simulink model "m04_linearization_model"  (R2021a)
settings: Solver=VariableStepAuto  StartTime=0.0  StopTime=10  RelTol=1e-3
undefined symbols (not defined in the file or in its folder): a, b, Cf, Cq, Cr, hs, Ix, Iz, Kq, M, ms
libraries: simulink x2
settings Model: Creator=jaime  LastModifiedBy=jaime

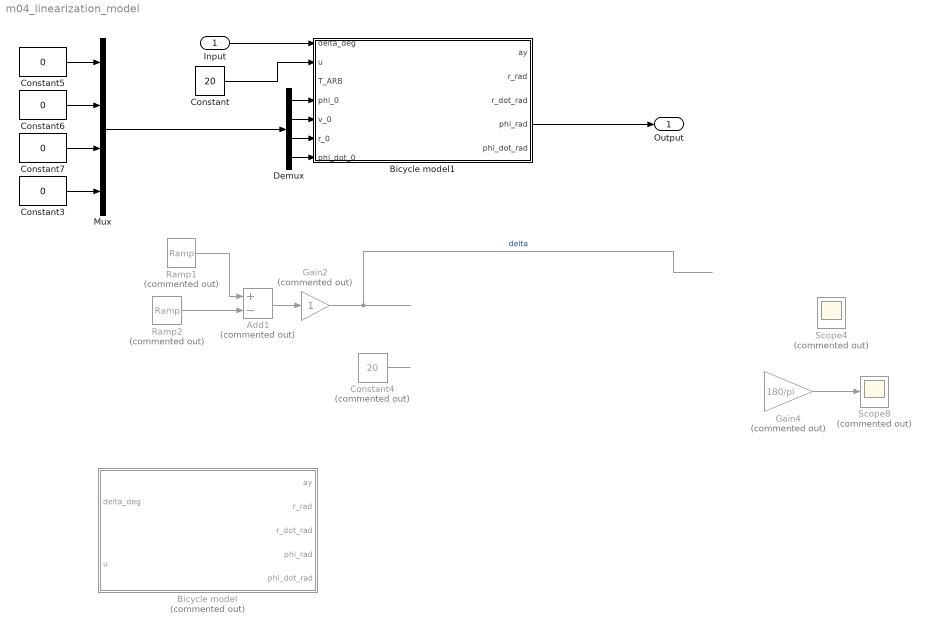
== system m04_linearization_model ==
  Input : Inport
  Add1 : Sum  Commented=on  Inputs=+-
  Bicycle model : Subsystem  Commented=on
  Bicycle model1 : Subsystem
  Constant : Constant  Value=20
  Constant{3,5..7} (4 alike) : Constant  Value=0
  Constant4 : Constant  Commented=on  Value=20
  Demux : Demux
  Gain2 : Gain  Commented=on
  Gain4 : Gain  Commented=on  Gain=180/pi
  Mux : Mux
  Ramp1 : simulink/Sources/Ramp  Commented=on  slope=2  start=0  InitialOutput=0
  Ramp2 : simulink/Sources/Ramp  Commented=on  slope=2  start=5  InitialOutput=0
  Scope4 : Scope  Commented=on  NumInputPorts=2
  Scope8 : Scope  Commented=on
  Output : Outport
  wires:
  Add1/1 -> Gain2/1
  Gain2/1 -> ?  "delta"
  Constant4/1 -> ?
  Ramp1/1 -> Add1/1
  Ramp2/1 -> Add1/2
  Gain4/1 -> Scope8/1
  ? -> Scope4/2  "ay"
  Input/1 -> Bicycle model1/1(delta_deg)
  Constant/1 -> Bicycle model1/2(u)
  Bicycle model1/4(phi_rad) -> Output/1
  Constant6/1 -> Mux/2
  Mux/1 -> Demux/1
  Constant7/1 -> Mux/3
  Constant5/1 -> Mux/1
  Constant3/1 -> Mux/4
  Demux/1 -> Bicycle model1/4(phi_0)
  Demux/2 -> Bicycle model1/5(v_0)
  Demux/3 -> Bicycle model1/6(r_0)
  Demux/4 -> Bicycle model1/7(phi_dot_0)

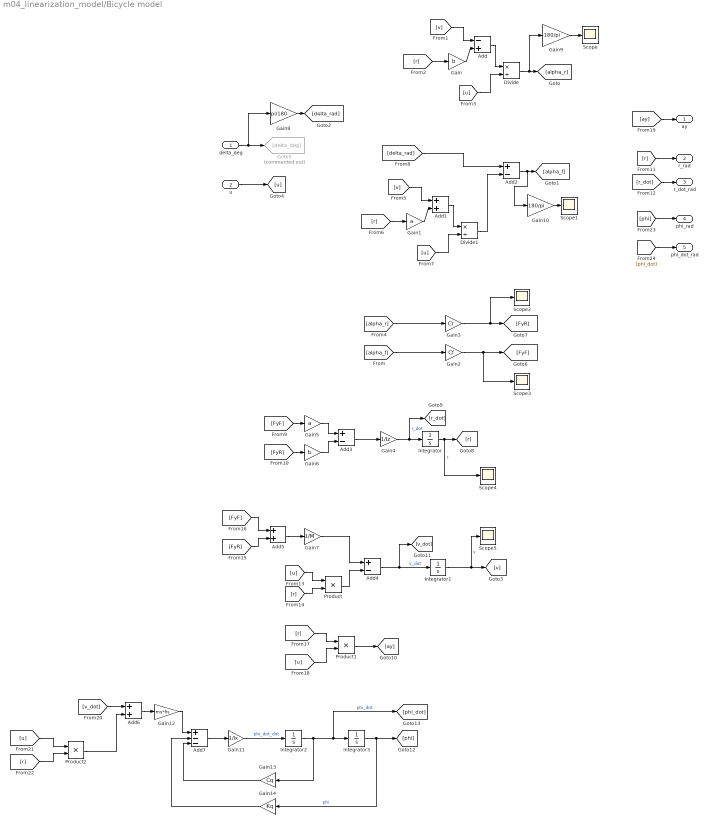
== system m04_linearization_model/Bicycle model ==
  delta_deg : Inport
  u : Inport  Port=2
  Add : Sum  Inputs=-+
  Add1 : Sum
  Add2 : Sum  Inputs=+-
  Add3 : Sum  Inputs=+-
  Add4 : Sum  Inputs=+-
  Add5 : Sum
  Add6 : Sum
  Add7 : Sum  Inputs=+--
  Divide : Product  Inputs=*/
  Divide1 : Product  Inputs=*/
  Gain : Gain  Gain=b
  Gain1 : Gain  Gain=a
  Gain10 : Gain  Gain=180/pi
  Gain11 : Gain  Gain=1/Ix
  Gain12 : Gain  Gain=ms*hs
  Gain13 : Gain  Gain=Cq
  Gain14 : Gain  Gain=Kq
  Gain2 : Gain  Gain=Cf
  Gain3 : Gain  Gain=Cr
  Gain4 : Gain  Gain=1/Iz
  Gain5 : Gain  Gain=a
  Gain6 : Gain  Gain=b
  Gain7 : Gain  Gain=1/M
  Gain8 : Gain  Gain=pi/180
  Gain9 : Gain  Gain=180/pi
  Goto5 : Goto  Commented=on  GotoTag=delta_deg
  Integrator{,1..3} (4 alike) : Integrator
  Product : Product
  Product1 : Product
  Product2 : Product
  Scope{,1..5} (6 alike) : Scope
  ay : Outport
  r_rad : Outport  Port=2
  r_dot_rad : Outport  Port=3
  phi_rad : Outport  Port=4
  phi_dot_rad : Outport  Port=5
  wires:
  [v] -> Add/1
  [r] -> Gain/1
  Gain/1 -> Add/2
  u/1 -> [u]
  [u] -> Divide/2
  Add/1 -> Divide/1
  Divide/1 -> Gain9/1, [alpha_r]
  Gain1/1 -> Add1/2
  Add1/1 -> Divide1/1
  [r] -> Gain1/1
  [v] -> Add1/1
  [u] -> Divide1/2
  Add2/1 -> Gain10/1, [alpha_f]
  delta_deg/1 -> Gain8/1, Goto5/1
  [delta_rad] -> Add2/1
  Divide1/1 -> Add2/2
  Gain3/1 -> Scope2/1, [FyR]
  Gain2/1 -> Scope3/1, [FyF]
  [alpha_r] -> Gain3/1
  [alpha_f] -> Gain2/1
  Integrator/1 -> Scope4/1, [r]  "r"
  Gain4/1 -> [r_dot], Integrator/1  "r_dot"
  [FyF] -> Gain5/1
  [FyR] -> Gain6/1
  Gain5/1 -> Add3/1
  Gain6/1 -> Add3/2
  Add3/1 -> Gain4/1
  [r] -> r_rad/1
  [r_dot] -> r_dot_rad/1
  Integrator1/1 -> Scope5/1, [v]  "v"
  Add4/1 -> [v_dot], Integrator1/1  "v_dot"
  [u] -> Product/1
  [r] -> Product/2
  Product/1 -> Add4/2
  [FyF] -> Add5/1
  [FyR] -> Add5/2
  Add5/1 -> Gain7/1
  Gain7/1 -> Add4/1
  [r] -> Product1/1
  [u] -> Product1/2
  Product1/1 -> [ay]
  [ay] -> ay/1
  Gain8/1 -> [delta_rad]
  Gain10/1 -> Scope1/1
  Gain9/1 -> Scope/1
  Integrator2/1 -> Gain13/1, [phi_dot], Integrator3/1  "phi_dot"
  Gain11/1 -> Integrator2/1  "phi_dot_dot"
  Integrator3/1 -> [phi], Gain14/1  "phi"
  [v_dot] -> Add6/1
  [u] -> Product2/1
  [r] -> Product2/2
  Product2/1 -> Add6/2
  Add6/1 -> Gain12/1
  Add7/1 -> Gain11/1
  Gain12/1 -> Add7/1
  Gain13/1 -> Add7/3
  Gain14/1 -> Add7/2
  [phi] -> phi_rad/1
  [phi_dot] -> phi_dot_rad/1

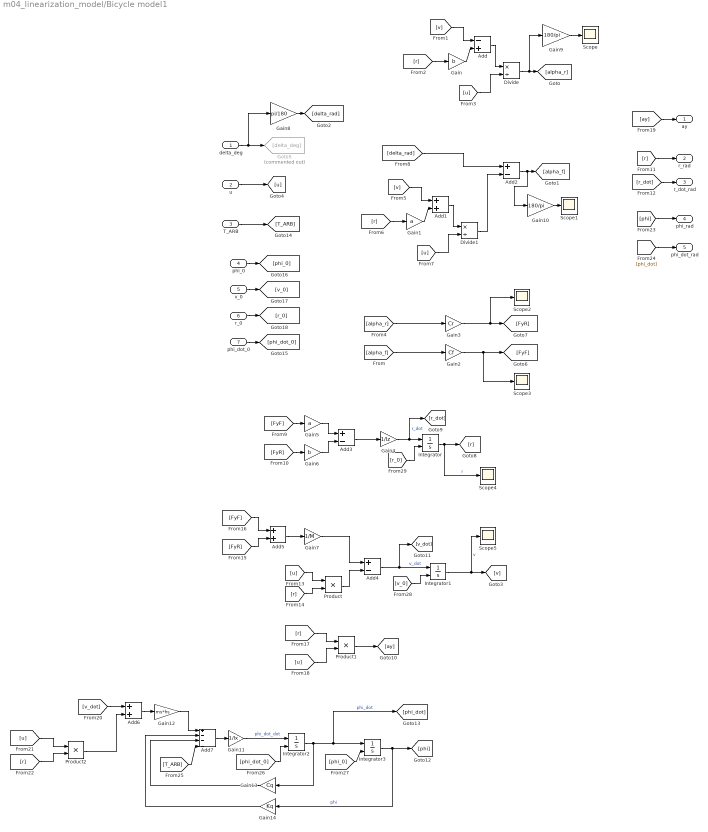
== system m04_linearization_model/Bicycle model1 ==
  delta_deg : Inport
  u : Inport  Port=2
  T_ARB : Inport  Port=3
  phi_0 : Inport  Port=4
  v_0 : Inport  Port=5
  r_0 : Inport  Port=6
  phi_dot_0 : Inport  Port=7
  Add : Sum  Inputs=-+
  Add1 : Sum
  Add2 : Sum  Inputs=+-
  Add3 : Sum  Inputs=+-
  Add4 : Sum  Inputs=+-
  Add5 : Sum
  Add6 : Sum
  Add7 : Sum  Inputs=+---
  Divide : Product  Inputs=*/
  Divide1 : Product  Inputs=*/
  Gain : Gain  Gain=b
  Gain1 : Gain  Gain=a
  Gain10 : Gain  Gain=180/pi
  Gain11 : Gain  Gain=1/Ix
  Gain12 : Gain  Gain=ms*hs
  Gain13 : Gain  Gain=Cq
  Gain14 : Gain  Gain=Kq
  Gain2 : Gain  Gain=Cf
  Gain3 : Gain  Gain=Cr
  Gain4 : Gain  Gain=1/Iz
  Gain5 : Gain  Gain=a
  Gain6 : Gain  Gain=b
  Gain7 : Gain  Gain=1/M
  Gain8 : Gain  Gain=pi/180
  Gain9 : Gain  Gain=180/pi
  Goto5 : Goto  Commented=on  GotoTag=delta_deg
  Integrator{,1..3} (4 alike) : Integrator  InitialConditionSource=external
  Product : Product
  Product1 : Product
  Product2 : Product
  Scope{,1..5} (6 alike) : Scope
  ay : Outport
  r_rad : Outport  Port=2
  r_dot_rad : Outport  Port=3
  phi_rad : Outport  Port=4
  phi_dot_rad : Outport  Port=5
  wires:
  [v] -> Add/1
  [r] -> Gain/1
  Gain/1 -> Add/2
  u/1 -> [u]
  [u] -> Divide/2
  Add/1 -> Divide/1
  Divide/1 -> Gain9/1, [alpha_r]
  Gain1/1 -> Add1/2
  Add1/1 -> Divide1/1
  [r] -> Gain1/1
  [v] -> Add1/1
  [u] -> Divide1/2
  Add2/1 -> Gain10/1, [alpha_f]
  delta_deg/1 -> Gain8/1, Goto5/1
  [delta_rad] -> Add2/1
  Divide1/1 -> Add2/2
  Gain3/1 -> Scope2/1, [FyR]
  Gain2/1 -> Scope3/1, [FyF]
  [alpha_r] -> Gain3/1
  [alpha_f] -> Gain2/1
  Integrator/1 -> [r], Scope4/1  "r"
  Gain4/1 -> [r_dot], Integrator/1  "r_dot"
  [FyF] -> Gain5/1
  [FyR] -> Gain6/1
  Gain5/1 -> Add3/1
  Gain6/1 -> Add3/2
  Add3/1 -> Gain4/1
  [r] -> r_rad/1
  [r_dot] -> r_dot_rad/1
  Integrator1/1 -> Scope5/1, [v]  "v"
  Add4/1 -> [v_dot], Integrator1/1  "v_dot"
  [u] -> Product/1
  [r] -> Product/2
  Product/1 -> Add4/2
  [FyF] -> Add5/1
  [FyR] -> Add5/2
  Add5/1 -> Gain7/1
  Gain7/1 -> Add4/1
  [r] -> Product1/1
  [u] -> Product1/2
  Product1/1 -> [ay]
  [ay] -> ay/1
  Gain8/1 -> [delta_rad]
  Gain10/1 -> Scope1/1
  Gain9/1 -> Scope/1
  Integrator2/1 -> [phi_dot], Integrator3/1, Gain13/1  "phi_dot"
  Gain11/1 -> Integrator2/1  "phi_dot_dot"
  Integrator3/1 -> [phi], Gain14/1  "phi"
  [v_dot] -> Add6/1
  [u] -> Product2/1
  [r] -> Product2/2
  Product2/1 -> Add6/2
  Add6/1 -> Gain12/1
  Add7/1 -> Gain11/1
  Gain12/1 -> Add7/1
  Gain13/1 -> Add7/3
  Gain14/1 -> Add7/2
  [phi] -> phi_rad/1
  [phi_dot] -> phi_dot_rad/1
  T_ARB/1 -> [T_ARB]
  [T_ARB] -> Add7/4
  [phi_dot_0] -> Integrator2/2
  [phi_0] -> Integrator3/2
  [v_0] -> Integrator1/2
  [r_0] -> Integrator/2
  v_0/1 -> [v_0]
  r_0/1 -> [r_0]
  phi_0/1 -> [phi_0]
  phi_dot_0/1 -> [phi_dot_0]
